simulink model "SimplifiedModel"  (R2022b)
settings: Solver=VariableStepAuto  StartTime=0.0  StopTime=500.0  RelTol=1e-3
settings Model: PacingRate=10  Creator=ADMIN  LastModifiedBy=ADMIN

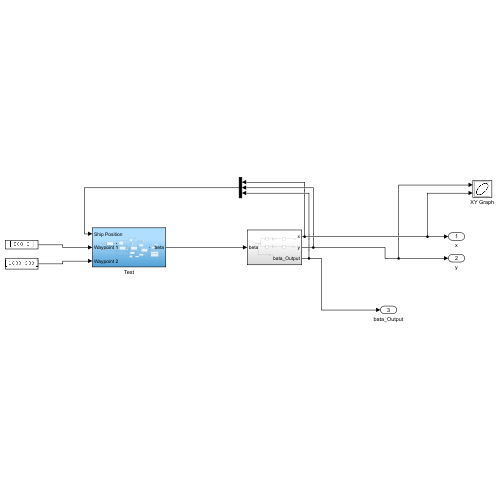
[thumbnail: Simulink's stored preview of the top-level diagram]
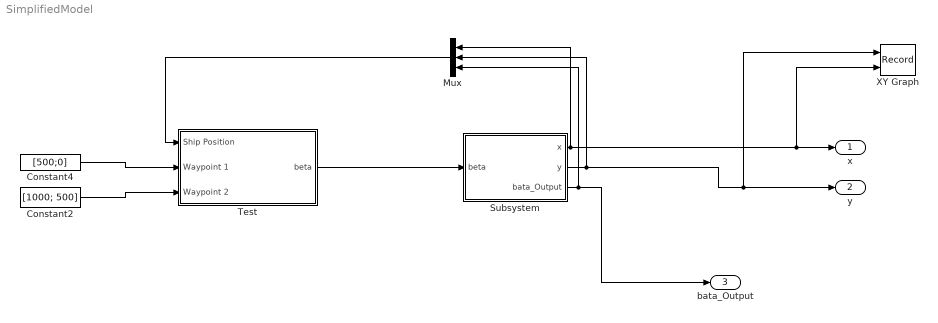
== system SimplifiedModel ==
  Constant2 : Constant  Value=[1000; 500]
  Constant4 : Constant  Value=[500;0]
  Mux : Mux  Inputs=3
  Subsystem : Subsystem
  Test : Subsystem
  XY Graph : Record  FileSettingsInternal="{\"entries\":[{\"content\":{\"excelSettings\":{\"content\":{},\"type\":\"Streamout.ExcelSettings\"}},\"type\":\"Streamout.FileSettingStorage\",\"uuid\":\"222b39a6-4560-418e-9ef3-1b49454d8de0\"}],\"packageUris\":[\"http://schema.mathworks.com/mf0/streamout_blocks/R2020a\"],\"version\":\"1.0\"}"  Layout=[1 1]  SignalsInternal="{\"entries\":[{\"content\":{\"signals\":[{\"content\":{\"blockPath\":[\"SimplifiedModel/XY Graph\"],\"channel\":[],\"dimensions\":[1],\"domain\":\"SimplifiedModel/XY Graph\",\"lineColor\":\"#a2142f\",\"plots\":[1],\"port\":1,\"sid\":[\"\"],\"signalID\":213,\"signalName\":\"Subsystem:2\"},\"type\":\"RecordBlkView.Signal\",\"uuid\":\"8755a672-e015-42b9-8710-c998a753ca6d\"},{\"content\":{\"blockPath\":[\"SimplifiedModel/XY Graph\"],\"channel\":[],\"dimensions\":[1],\"domain\":\"SimplifiedModel/XY Graph\",\"lineColor\":\"#139fff\",\"plots\":[1],\"port\":2,\"sid\":[\"\"],\"signalID\":217,\"signalName\":\"Subsystem:1\"},\"type\":\"RecordBlkView.Signal\",\"uuid\":\"ba0069ad-23bc-4acb-b8d1-cdf852fc7748\"}]},\"type\":\"RecordBlkView.InputSignals\",\"uuid\":\"6c1eb284-240b-4263-8c83-bd05b5197710\"}],\"packageUris\":[\"http://schema.mathworks.com/mf0/streamout_blocks/R2020a\"],\"version\":\"1.0\"}"  VisualizationBindings="{\"xyplotplugin\":{\"info\":[{\"series\":[{\"bindingParametersList\":[{\"parameter\":\"X-Axis\",\"signalID\":213,\"signalName\":\"Subsystem:2\"},{\"parameter\":\"Y-Axis\",\"signalID\":217,\"signalName\":\"Subsystem:1\"}],\"seriesID\":1047}],\"subplotID\":1}]}}"  CompatibilityTag=XY
  x : Outport
  y : Outport  Port=2
  bata_Output : Outport  Port=3
  wires:
  Subsystem/1(x) -> Mux/1, XY Graph/2, x/1
  Subsystem/2(y) -> Mux/2, XY Graph/1, y/1
  Subsystem/3(bata_Output) -> Mux/3, bata_Output/1
  Constant2/1 -> Test/3(Waypoint 2)
  Constant4/1 -> Test/2(Waypoint 1)
  Test/1(beta) -> Subsystem/1(beta)
  Mux/1 -> Test/1(Ship Position)

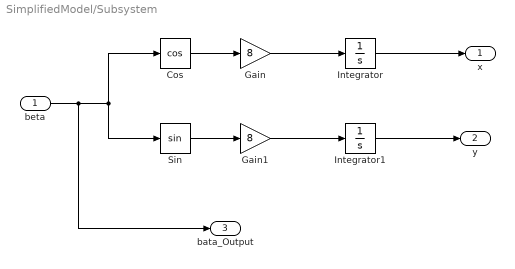
== system SimplifiedModel/Subsystem ==
  beta : Inport
  Cos : Trigonometry  Operator=cos
  Gain : Gain  Gain=8
  Gain1 : Gain  Gain=8
  Integrator : Integrator
  Integrator1 : Integrator
  Sin : Trigonometry
  x : Outport
  y : Outport  Port=2
  bata_Output : Outport  Port=3
  wires:
  Sin/1 -> Gain1/1
  Integrator1/1 -> y/1
  Gain/1 -> Integrator/1
  beta/1 -> bata_Output/1, Cos/1, Sin/1
  Cos/1 -> Gain/1
  Integrator/1 -> x/1
  Gain1/1 -> Integrator1/1

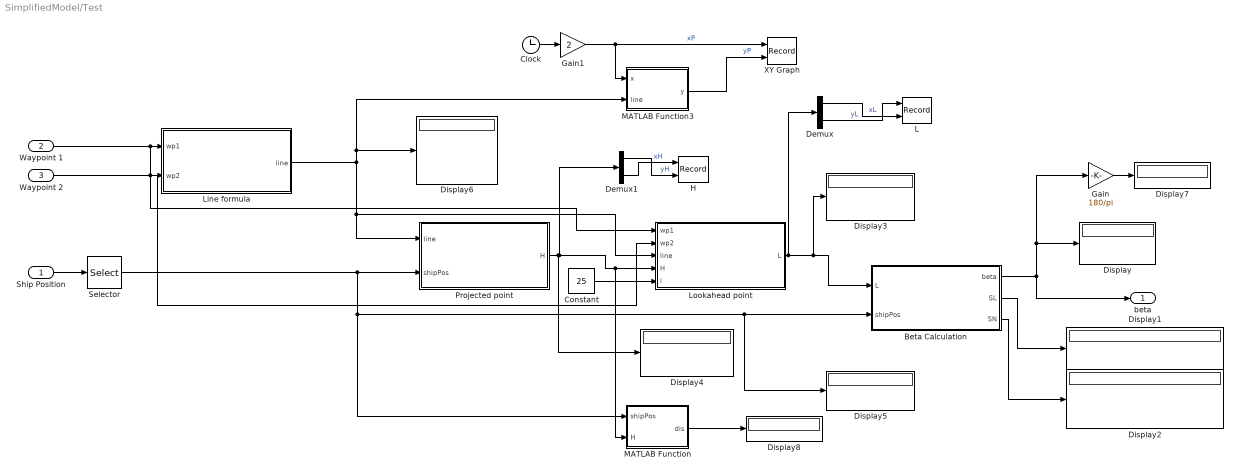
== system SimplifiedModel/Test ==
  Ship Position : Inport
  Waypoint 1 : Inport  Port=2
  Waypoint 2 : Inport  Port=3
  Beta Calculation : MATLAB Function  TreatAsAtomicUnit=on
  Clock : Clock
  Constant : Constant  Value=25
  Demux : Demux  Outputs=2
  Demux1 : Demux  Outputs=2
  Display{,1..8} (9 alike) : Display
  Gain : Gain  Gain=180/pi
  Gain1 : Gain  Gain=2
  H : Record  FileSettingsInternal="{\"entries\":[{\"content\":{\"excelSettings\":{\"content\":{},\"type\":\"Streamout.ExcelSettings\"}},\"type\":\"Streamout.FileSettingStorage\",\"uuid\":\"acb4f9e4-790d-4f81-af84-a0ca8f65199c\"}],\"packageUris\":[\"http://schema.mathworks.com/mf0/streamout_blocks/R2020a\"],\"version\":\"1.0\"}"  Layout=[1 1]  SignalsInternal="{\"entries\":[{\"content\":{\"signals\":[{\"content\":{\"blockPath\":[\"SimplifiedModel/Test/H\"],\"channel\":[],\"dimensions\":[1,1],\"domain\":\"SimplifiedModel/Test/H\",\"lineColor\":\"#64d413\",\"plots\":[1],\"port\":1,\"sid\":[\"\"],\"signalID\":221,\"signalName\":\"xH\"},\"type\":\"RecordBlkView.Signal\",\"uuid\":\"73abfa25-c011-4411-b49e-7aad8b0877a7\"},{\"content\":{\"blockPath\":[\"SimplifiedModel/Test/H\"],\"channel\":[],\"dimensions\":[1,1],\"domain\":\"SimplifiedModel/Test/H\",\"lineColor\":\"#ff13a6\",\"plots\":[1],\"port\":2,\"sid\":[\"\"],\"signalID\":225,\"signalName\":\"yH\"},\"type\":\"RecordBlkView.Signal\",\"uuid\":\"31bb5b4d-afc9-4333-b8f6-2635f36eda98\"}]},\"type\":\"RecordBlkView.InputSignals\",\"uuid\":\"61b53e87-936c-468d-a2b8-1f96c0468e4d\"}],\"packageUris\":[\"http://schema.mathworks.com/mf0/streamout_blocks/R2020a\"],\"version\":\"1.0\"}"  VisualizationBindings="{\"xyplotplugin\":{\"info\":[{\"series\":[{\"bindingParametersList\":[{\"parameter\":\"X-Axis\",\"signalID\":221,\"signalName\":\"xH\"},{\"parameter\":\"Y-Axis\",\"signalID\":225,\"signalName\":\"yH\"}],\"seriesID\":20278}],\"subplotID\":1}]}}"  CompatibilityTag=XY
  L : Record  FileSettingsInternal="{\"entries\":[{\"content\":{\"excelSettings\":{\"content\":{},\"type\":\"Streamout.ExcelSettings\"}},\"type\":\"Streamout.FileSettingStorage\",\"uuid\":\"e508f10e-f8bc-4f73-9880-21389b8213aa\"}],\"packageUris\":[\"http://schema.mathworks.com/mf0/streamout_blocks/R2020a\"],\"version\":\"1.0\"}"  Layout=[1 1]  SignalsInternal="{\"entries\":[{\"content\":{\"signals\":[{\"content\":{\"blockPath\":[\"SimplifiedModel/Test/L\"],\"channel\":[],\"dimensions\":[1,1],\"domain\":\"SimplifiedModel/Test/L\",\"lineColor\":\"#64d413\",\"plots\":[1],\"port\":1,\"sid\":[\"\"],\"signalID\":229,\"signalName\":\"yL\"},\"type\":\"RecordBlkView.Signal\",\"uuid\":\"32b916f2-9a90-4b41-93bb-334b34aadc40\"},{\"content\":{\"blockPath\":[\"SimplifiedModel/Test/L\"],\"channel\":[],\"dimensions\":[1,1],\"domain\":\"SimplifiedModel/Test/L\",\"lineColor\":\"#ff13a6\",\"plots\":[1],\"port\":2,\"sid\":[\"\"],\"signalID\":233,\"signalName\":\"xL\"},\"type\":\"RecordBlkView.Signal\",\"uuid\":\"b26a90b1-bbab-4bd0-81b9-26254e4924f2\"}]},\"type\":\"RecordBlkView.InputSignals\",\"uuid\":\"fe685b2e-f0fc-4860-b782-313dd8c3d872\"}],\"packageUris\":[\"http://schema.mathworks.com/mf0/streamout_blocks/R2020a\"],\"version\":\"1.0\"}"  VisualizationBindings="{\"xyplotplugin\":{\"info\":[{\"series\":[{\"bindingParametersList\":[{\"parameter\":\"X-Axis\",\"signalID\":229,\"signalName\":\"yL\"},{\"parameter\":\"Y-Axis\",\"signalID\":233,\"signalName\":\"xL\"}],\"seriesID\":18917}],\"subplotID\":1}]}}"  CompatibilityTag=XY
  Line formula : MATLAB Function  TreatAsAtomicUnit=on
  Lookahead point : MATLAB Function  TreatAsAtomicUnit=on
  MATLAB Function : MATLAB Function  TreatAsAtomicUnit=on
  MATLAB Function3 : MATLAB Function  TreatAsAtomicUnit=on
  Projected point : MATLAB Function  TreatAsAtomicUnit=on
  Selector : Selector  InputPortWidth=3  IndexOptions=Index vector (dialog)  Indices=[1 2]  OutputSizes=1
  XY Graph : Record  FileSettingsInternal="{\"entries\":[{\"content\":{\"excelSettings\":{\"content\":{},\"type\":\"Streamout.ExcelSettings\"}},\"type\":\"Streamout.FileSettingStorage\",\"uuid\":\"c79b6d77-ece6-4ec3-b944-a9e8fdf4f102\"}],\"packageUris\":[\"http://schema.mathworks.com/mf0/streamout_blocks/R2020a\"],\"version\":\"1.0\"}"  Layout=[1 1]  SignalsInternal="{\"entries\":[{\"content\":{\"signals\":[{\"content\":{\"blockPath\":[\"SimplifiedModel/Test/XY Graph\"],\"channel\":[],\"dimensions\":[1],\"domain\":\"SimplifiedModel/Test/XY Graph\",\"lineColor\":\"#64d413\",\"plots\":[1],\"port\":1,\"sid\":[\"\"],\"signalID\":237,\"signalName\":\"xP\"},\"type\":\"RecordBlkView.Signal\",\"uuid\":\"3cbeaab6-5ceb-4126-b36f-4828747ea49f\"},{\"content\":{\"blockPath\":[\"SimplifiedModel/Test/XY Graph\"],\"channel\":[],\"dimensions\":[1],\"domain\":\"SimplifiedModel/Test/XY Graph\",\"lineColor\":\"#ff13a6\",\"plots\":[1],\"port\":2,\"sid\":[\"\"],\"signalID\":241,\"signalName\":\"yP\"},\"type\":\"RecordBlkView.Signal\",\"uuid\":\"5af3af22-ebed-4a58-bd62-5a9be8efd216\"}]},\"type\":\"RecordBlkView.InputSignals\",\"uuid\":\"656978a9-75c9-4c0e-8c6b-1e47793a6008\"}],\"packageUris\":[\"http://schema.mathworks.com/mf0/streamout_blocks/R2020a\"],\"version\":\"1.0\"}"  VisualizationBindings="{\"xyplotplugin\":{\"info\":[{\"series\":[{\"bindingParametersList\":[{\"parameter\":\"X-Axis\",\"signalID\":237,\"signalName\":\"xP\"},{\"parameter\":\"Y-Axis\",\"signalID\":241,\"signalName\":\"yP\"}],\"seriesID\":33402}],\"subplotID\":1}]}}"  CompatibilityTag=XY
  beta : Outport
  wires:
  Waypoint 1/1 -> Lookahead point/1(wp1), Line formula/1(wp1)
  Waypoint 2/1 -> Lookahead point/2(wp2), Line formula/2(wp2)
  Ship Position/1 -> Selector/1
  Projected point/1(H) -> Display4/1, Demux1/1, MATLAB Function/2(H), Lookahead point/4(H)
  Constant/1 -> Lookahead point/5(l)
  Lookahead point/1(L) -> Demux/1, Display3/1, Beta Calculation/1(L)
  Beta Calculation/1(beta) -> beta/1, Display/1, Gain/1
  Beta Calculation/2(SL) -> Display1/1
  Beta Calculation/3(SN) -> Display2/1
  Selector/1 -> Display5/1, Beta Calculation/2(shipPos), MATLAB Function/1(shipPos), Projected point/2(shipPos)
  Gain/1 -> Display7/1
  Gain1/1 -> XY Graph/1, MATLAB Function3/1(x)  "xP"
  Clock/1 -> Gain1/1
  Line formula/1(line) -> Lookahead point/3(line), Projected point/1(line), MATLAB Function3/2(line), Display6/1
  MATLAB Function3/1(y) -> XY Graph/2  "yP"
  Demux/1 -> L/2  "xL"
  Demux/2 -> L/1  "yL"
  Demux1/1 -> H/2  "yH"
  Demux1/2 -> H/1  "xH"
  MATLAB Function/1(dis) -> Display8/1

== matlab function SimplifiedModel/Test/Beta Calculation ==
  data: L input; beta output; shipPos input; SL output; SN output
function [beta, SL, SN] = fcn(L, shipPos)

N = shipPos' + [0 500]; % arbitrary point on the North axis of the ship
SL = L - shipPos'; % lookahead vector
SN = N - shipPos'; % North vector
beta = acos(dot(SL, SN) / (norm(SL) * norm(SN))); % angle between 2 vectors

% Determine correct sign for beta
if L(1) < shipPos(1)
   beta = -beta;
end

== matlab function SimplifiedModel/Test/Line formula ==
  data: wp1 input; line output; wp2 input
function line = fcn(wp1, wp2)

% Reverse coordinate of points
wayPoint1 = flip(wp1);
wayPoint2 = flip(wp2);

a = (wayPoint2(1) - wayPoint1(1)) / (wayPoint2(2) - wayPoint1(2));
b = -1;
c = wayPoint1(2) - a*wayPoint1(1);

line = [a, b, c];
% ax + by + c = 0

== matlab function SimplifiedModel/Test/Lookahead point ==
  data: wp1 input; wp2 input; line input; L output; H input; l input
function L = fcn(wp1, wp2, line, H, l)
lineFormula = line;
projectedPoint = H;
distance = l;
coder.extrinsic('LookAhead');
L = [0 0];
L = LookAhead(wp1, wp2, line, H, l);

== matlab function SimplifiedModel/Test/Projected point ==
  data: line input; H output; shipPos input
function H = fcn(line, shipPos) 
coder.extrinsic('PointProjection');
H = [0, 0];
H = PointProjection(shipPos, line);

== matlab function SimplifiedModel/Test/MATLAB Function3 ==
  data: x input; y output; line input
function y = fcn(x,line)

y = line(1)*x+line(3);

== matlab function SimplifiedModel/Test/MATLAB Function ==
  data: shipPos input; dis output; H input
function dis = fcn(shipPos, H)

dis = sqrt( (shipPos(1)-H(1))^2 + (shipPos(2)-H(2))^2);
